simulink model "Lab_07_QPSK_Modulation_and_Demodulation_Simulink_Lab"  (R2018a)
settings: Solver=VariableStepAuto  StartTime=0.0  StopTime=10.0  RelTol=1e-3
libraries: commutil2 x4, dspsrcs4 x4, commrandsrc3 x2, commfilt2 x2, simulink x2
settings Model: Creator=m_nou  LastModifiedBy=m_nou

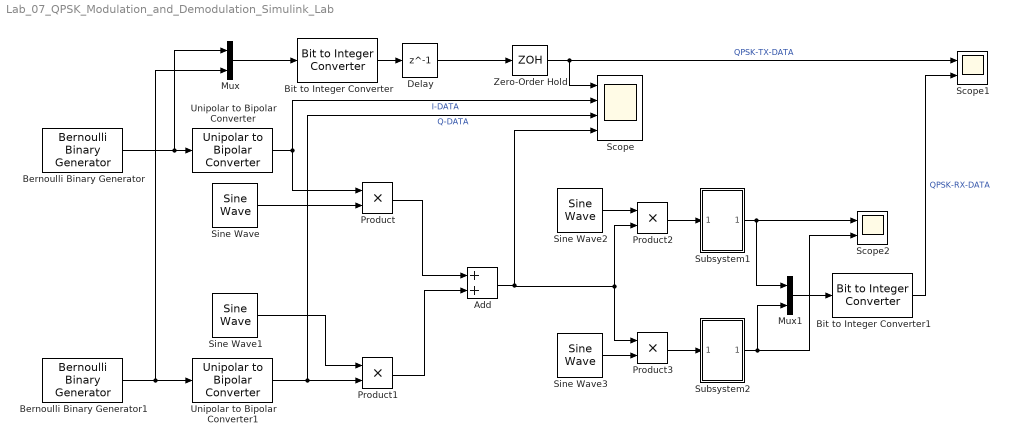
== system Lab_07_QPSK_Modulation_and_Demodulation_Simulink_Lab ==
  Add : Sum
  Bernoulli Binary Generator : commrandsrc3/Bernoulli Binary Generator  ProbabilityOfZero=0.5  SeedSource=Auto  Seed=0  SampleTime=1  SamplesPerFrame=1  OutputDataType=double  SimulateUsing=Interpreted execution
  Bernoulli Binary Generator1 : commrandsrc3/Bernoulli Binary Generator  ProbabilityOfZero=0.5  SeedSource=Auto  Seed=0  SampleTime=1  SamplesPerFrame=1  OutputDataType=double  SimulateUsing=Interpreted execution
  Bit to Integer Converter : commutil2/Bit to Integer Converter  nbits=2  bitOrder=MSB first  signedOutputValues=Unsigned  outDtype=Inherit via internal rule  outDtypeSigned=Inherit via internal rule
  Bit to Integer Converter1 : commutil2/Bit to Integer Converter  nbits=2  bitOrder=MSB first  signedOutputValues=Unsigned  outDtype=Inherit via internal rule  outDtypeSigned=Inherit via internal rule
  Delay : Delay  DelayLength=1  InitialCondition=0
  Mux : Mux  Inputs=2
  Mux1 : Mux  Inputs=2
  Product{,1..3} (4 alike) : Product
  Scope : Scope  NumInputPorts=4
  Scope1 : Scope  NumInputPorts=2
  Scope2 : Scope  NumInputPorts=2
  Sine Wave : dspsrcs4/Sine Wave  Amplitude=1  Frequency=5  Phase=0  SampleMode=Discrete  OutComplex=Real  CompMethod=Trigonometric fcn  TableSize=Speed  SampleTime=1/100  SamplesPerFrame=1  ResetState=Restart at time zero  OutputFrames=off  dataType=double  wordLen=16  udDataType=sfix(16)  fracBitsMode=Best precision  numFracBits=15  OutDataTypeStr=double  LastOutDataTypeStr=double
  Sine Wave1 : dspsrcs4/Sine Wave  Amplitude=1  Frequency=5  Phase=pi/2  SampleMode=Discrete  OutComplex=Real  CompMethod=Trigonometric fcn  TableSize=Speed  SampleTime=1/100  SamplesPerFrame=1  ResetState=Restart at time zero  OutputFrames=off  dataType=double  wordLen=16  udDataType=sfix(16)  fracBitsMode=Best precision  numFracBits=15  OutDataTypeStr=double  LastOutDataTypeStr=double
  Sine Wave2 : dspsrcs4/Sine Wave  Amplitude=1  Frequency=5  Phase=0  SampleMode=Discrete  OutComplex=Real  CompMethod=Trigonometric fcn  TableSize=Speed  SampleTime=1/100  SamplesPerFrame=1  ResetState=Restart at time zero  OutputFrames=off  dataType=double  wordLen=16  udDataType=sfix(16)  fracBitsMode=Best precision  numFracBits=15  OutDataTypeStr=double  LastOutDataTypeStr=double
  Sine Wave3 : dspsrcs4/Sine Wave  Amplitude=1  Frequency=5  Phase=pi/2  SampleMode=Discrete  OutComplex=Real  CompMethod=Trigonometric fcn  TableSize=Speed  SampleTime=1/100  SamplesPerFrame=1  ResetState=Restart at time zero  OutputFrames=off  dataType=double  wordLen=16  udDataType=sfix(16)  fracBitsMode=Best precision  numFracBits=15  OutDataTypeStr=double  LastOutDataTypeStr=double
  Subsystem1 : Subsystem
  Subsystem2 : Subsystem
  Unipolar to Bipolar Converter : commutil2/Unipolar to Bipolar Converter  M=2  polarity=Positive  dataType=Inherit via internal rule
      settings: SourceProductName=Communications System Toolbox
  Unipolar to Bipolar Converter1 : commutil2/Unipolar to Bipolar Converter  M=2  polarity=Positive  dataType=Inherit via internal rule
      settings: SourceProductName=Communications System Toolbox
  Zero-Order Hold : ZeroOrderHold  SampleTime=-1
  wires:
  Sine Wave/1 -> Product/2
  Bit to Integer Converter/1 -> Delay/1
  Mux/1 -> Bit to Integer Converter/1
  Sine Wave2/1 -> Product2/1
  Sine Wave3/1 -> Product3/2
  Add/1 -> Scope/4, Product2/2, Product3/1
  Mux1/1 -> Bit to Integer Converter1/1
  Bit to Integer Converter1/1 -> Scope1/2  "QPSK-RX-DATA"
  Product2/1 -> Subsystem1/1(In1)
  Product3/1 -> Subsystem2/1(In1)
  Delay/1 -> Zero-Order Hold/1
  Zero-Order Hold/1 -> Scope1/1, Scope/1  "QPSK-TX-DATA"
  Product/1 -> Add/1
  Product1/1 -> Add/2
  Bernoulli Binary Generator1/1 -> Mux/2, Unipolar to Bipolar Converter1/1
  Unipolar to Bipolar Converter/1 -> Scope/2, Product/1  "I-DATA"
  Sine Wave1/1 -> Product1/1
  Subsystem1/1(Out1) -> Scope2/1, Mux1/1
  Subsystem2/1(Out1) -> Scope2/2, Mux1/2
  Unipolar to Bipolar Converter1/1 -> Product1/2, Scope/3  "Q-DATA"
  Bernoulli Binary Generator/1 -> Mux/1, Unipolar to Bipolar Converter/1

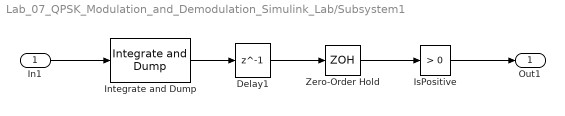
== system Lab_07_QPSK_Modulation_and_Demodulation_Simulink_Lab/Subsystem1 ==
  In1 : Inport
  Delay1 : Delay  DelayLength=1  InitialCondition=0
  Integrate and Dump : commfilt2/Integrate and Dump  obssamples=100  offsetsamples=0  nodump=off  roundingMode=Floor  overflowMode=off  outputDataTypeStr=Inherit: Same as accumulator  outputLastDataTypeStr=Inherit: Same as accumulator
      settings: SourceProductName=Communications System Toolbox
  IsPositive : simulink/Logic and Bit Operations/Compare To Zero  relop=>  OutDataTypeStr=boolean
  Zero-Order Hold : ZeroOrderHold  SampleTime=-1
  Out1 : Outport
  wires:
  Zero-Order Hold/1 -> IsPositive/1
  In1/1 -> Integrate and Dump/1
  Integrate and Dump/1 -> Delay1/1
  IsPositive/1 -> Out1/1
  Delay1/1 -> Zero-Order Hold/1

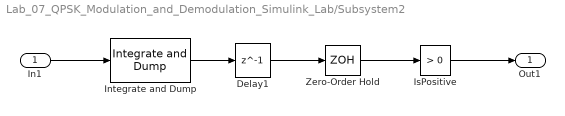
== system Lab_07_QPSK_Modulation_and_Demodulation_Simulink_Lab/Subsystem2 ==
  In1 : Inport
  Delay1 : Delay  DelayLength=1  InitialCondition=0
  Integrate and Dump : commfilt2/Integrate and Dump  obssamples=100  offsetsamples=0  nodump=off  roundingMode=Floor  overflowMode=off  outputDataTypeStr=Inherit: Same as accumulator  outputLastDataTypeStr=Inherit: Same as accumulator
      settings: SourceProductName=Communications System Toolbox
  IsPositive : simulink/Logic and Bit Operations/Compare To Zero  relop=>  OutDataTypeStr=boolean
  Zero-Order Hold : ZeroOrderHold  SampleTime=-1
  Out1 : Outport
  wires:
  Zero-Order Hold/1 -> IsPositive/1
  In1/1 -> Integrate and Dump/1
  Integrate and Dump/1 -> Delay1/1
  IsPositive/1 -> Out1/1
  Delay1/1 -> Zero-Order Hold/1
